simulink model "task3_lab11"  (R2021a)
settings: Solver=VariableStepAuto  StartTime=0.0  StopTime=10.0  RelTol=1e-3
libraries: simulink x1
settings Model: Creator=reemb  LastModifiedBy=reemb

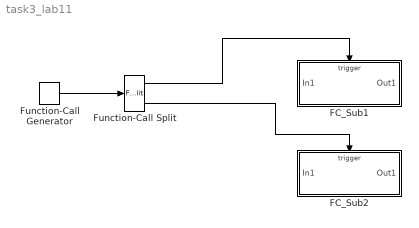
== system task3_lab11 ==
  FC_Sub1 : Subsystem  TreatAsAtomicUnit=on
  FC_Sub2 : Subsystem  TreatAsAtomicUnit=on
  Function-Call Generator : simulink/Ports & Subsystems/Function-Call Generator  sample_time=0.5  numberOfIterations=1  DisallowWideOutput=off
  Function-Call Split : FunctionCallSplit  IconShape=distinctive  NumOutputPorts=2  OutputPortLayout=default
  wires:
  Function-Call Generator/1 -> Function-Call Split/1
  Function-Call Split/1 -> FC_Sub1/Trigger
  Function-Call Split/2 -> FC_Sub2/Trigger

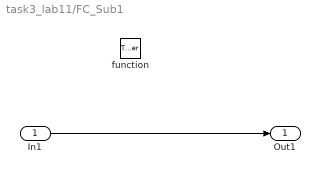
== system task3_lab11/FC_Sub1 ==
  In1 : Inport
  function : TriggerPort  TriggerType=function-call  VariantControl=(inherit)
  Out1 : Outport
  wires:
  In1/1 -> Out1/1

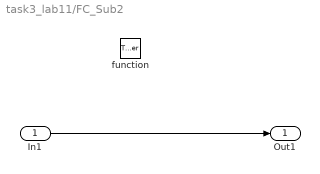
== system task3_lab11/FC_Sub2 ==
  In1 : Inport
  function : TriggerPort  TriggerType=function-call  VariantControl=(inherit)
  Out1 : Outport
  wires:
  In1/1 -> Out1/1
